simulink model "pdex"  (Simulink 8.5)
settings: Solver=ode45  SolverMode=SingleTasking  StartTime=0.0  StopTime=1.0  RelTol=1e-3  AbsTol=1e-6
libraries: tools x1, simulink x1
settings Model: Creator=PC  LastModifiedBy=PC
settings DataIOCC: LimitDataPoints=off
settings OptimizationCC: BlockReduction=off  BooleanDataType=off  ExpressionDepthLimit=128
settings DebuggingCC: SaveWithParameterizedLinksMsg=none  SignalResolutionControl=TryResolveAllWithWarning  MultiTaskDSMMsg=warning  MultiTaskCondExecSysMsg=none  FcnCallInpInsideContextMsg=EnableAllAsError  StateNameClashWarn=none
settings HardwareCC: TargetUnknown=on

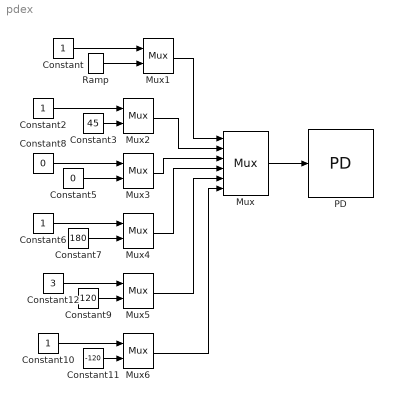
== system pdex ==
  Constant{,2,6,10} (4 alike) : Constant
  Constant11 : Constant  Value=-120
  Constant12 : Constant  Value=3
  Constant3 : Constant  Value=45
  Constant5 : Constant  Value=0
  Constant7 : Constant  Value=180
  Constant8 : Constant  Value=0
  Constant9 : Constant  Value=120
  Mux : Mux  Inputs=6
  Mux{1..6} (6 alike) : Mux  Inputs=2
  PD : tools/PD  Bactive=on  type=transient  dint=0.1
  Ramp : simulink/Sources/Ramp  slope=360  start=0  X0=0
  wires:
  Constant/1 -> Mux1/1
  Ramp/1 -> Mux1/2
  Constant2/1 -> Mux2/1
  Constant3/1 -> Mux2/2
  Constant6/1 -> Mux4/1
  Constant7/1 -> Mux4/2
  Constant12/1 -> Mux5/1
  Constant9/1 -> Mux5/2
  Constant10/1 -> Mux6/1
  Constant11/1 -> Mux6/2
  Mux1/1 -> Mux/1
  Mux2/1 -> Mux/2
  Mux3/1 -> Mux/3
  Mux4/1 -> Mux/4
  Mux5/1 -> Mux/5
  Mux6/1 -> Mux/6
  Constant8/1 -> Mux3/1
  Constant5/1 -> Mux3/2
  Mux/1 -> PD/1
